simulink model "PuenteH_dcdc_CUESTION2"  (R2024b)
settings: Solver=ode23s  StartTime=0.0  StopTime=Ts*nciclos  FixedStep=fixedstep  MaxStep=Ts/ssamples  RelTol=Auto  AbsTol=1e-3
InitFcn:
  | Ts=1/fs;
values from neighbouring files (symbols this model uses):
  fs = 10e3    (= 10000)    [Cuestion2.m]    (also in DatosBasePuenteH.m)
  seleccion = 2    [Cuestion2.m]
  ssamples = 200    [Cuestion2.m]    (also in DatosBasePuenteH.m)
  Vcont = 2*D - 1    [Cuestion2.m]    (also in DatosBasePuenteH.m = -0.6)
libraries: simulink x2, spsMultimeterLib x2, spsControlledCurrentSourceLib x1, spsDCVoltageSourceLib x1, spsOnDelayLib x1, spsUniversalBridgeLib x1, spsVoltageMeasurementLib x1, sps_lib x1
settings Model: Creator=patrice  LastModifiedBy=Pablo
settings SolverCC: AutoScaleAbsTol=off  AlgebraicLoopSolver=TrustRegion
settings DataIOCC: SaveFormat=StructureWithTime  SignalLoggingSaveFormat=ModelDataLogs  ReturnWorkspaceOutputs=off  TimeSaveName=tiempo  SignalLoggingName=sigsOut
settings OptimizationCC: BlockReduction=off  BooleanDataType=off  ExpressionDepthLimit=2147483647  InitFltsAndDblsToZero=on  LifeSpan=inf
settings DebuggingCC: SaveWithParameterizedLinksMsg=none  UnderspecifiedInitializationDetection=Classic  MergeDetectMultiDrivingBlocksExec=none  SignalResolutionControl=TryResolveAllWithWarning  MultiTaskDSMMsg=warning  MultiTaskCondExecSysMsg=none  FcnCallInpInsideContextMsg=warning  StateNameClashWarn=warning  SFUnexpectedBacktrackingDiag=warning  SFNoUnconditionalDefaultTransitionDiag=warning  SFExecutionAtInitializationDiag=none  ArithmeticOperatorsInVariantConditions=warning
settings HardwareCC: ProdBitPerPointer=32  ProdBitPerSizeT=32  ProdBitPerPtrDiffT=32  ProdLargestAtomicFloat=None  ProdIntDivRoundTo=Undefined  ProdEndianess=Unspecified  ProdWordSize=32  ProdHWDeviceType=32-bit Generic  TargetUnknown=on
settings ModelReferenceCC: EnableRefExpFcnMdlSchedulingChecks=on  PropagateSignalLabelsOutOfModel=off
settings SFSimCC: SimUseLocalCustomCode=off  CustomCodeUndefinedFunction=UseInterfaceOnly
settings RTWCC: TemplateMakefile=grt_unix.tmf  RTWUseLocalCustomCode=off  GPUComputeCapability=3.5  DLArmComputeVersion=19.05
settings CodeAppCC: StateflowObjectComments=on
settings GRTTargetCC: TargetFcnLib=ansi_tfl_tmw.mat  TargetLangStandard=C89/C90 (ANSI)  CombineOutputUpdateFcns=off  GRTInterface=on
settings ConfigComp: CovMetricSettings=dw  CovSaveCumulativeToWorkspaceVar=on  CovSaveSingleToWorkspaceVar=on  CovExternalEMLEnable=off
settings SimscapeCC: SimscapeNormalizeSystem=off

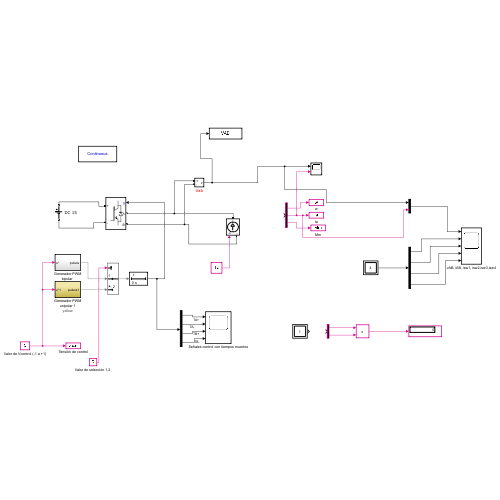
[thumbnail: Simulink's stored preview of the top-level diagram]
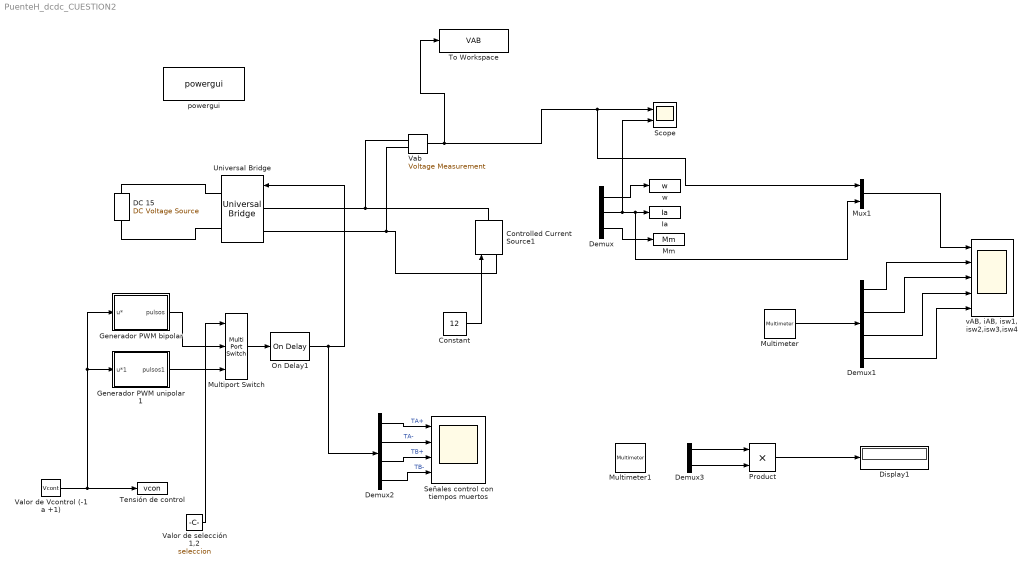
== system PuenteH_dcdc_CUESTION2 ==
  Constant : Constant  Value=12
  Controlled Current Source1 : spsControlledCurrentSourceLib/Controlled Current Source  Initialize=on  Source_Type=DC  Amplitude=12  Phase=0  Frequency=0  Measurements=Current
  DC 15 : spsDCVoltageSourceLib/DC Voltage Source  Amplitude=15  Measurements=Voltage
  Demux : Demux  Outputs=3
      settings: DisplayOption=none
  Demux1 : Demux
  Demux2 : Demux
  Demux3 : Demux  Outputs=2
  Display1 : Display
  "Generador PWM bipolar " : Subsystem
  Generador PWM unipolar 1 : Subsystem
      settings: AttributesFormatString=%<BackgroundColor>
  Ia : ToWorkspace  VariableName=Ia  SampleTime=-1
  Mm : ToWorkspace  VariableName=Mm  SampleTime=-1
  Multimeter : spsMultimeterLib/Multimeter  L=12  sel=[8 9 10 11]  yselected={}  Gain=[1 1 1 1]  OutputType=Complex  PlotAtSimulationStop=off  PhasorSimulation=off
  Multimeter1 : spsMultimeterLib/Multimeter  L=12  sel=7  yselected={}  Gain=1  OutputType=Complex  PlotAtSimulationStop=off  PhasorSimulation=off
  Multiport Switch : MultiPortSwitch  Inputs=2  SaturateOnIntegerOverflow=off  InputSameDT=off
  Mux1 : Mux  Inputs=2
  On Delay1 : spsOnDelayLib/On Delay  DelayType=On delay  delay=Tmuertos  ic=0  Ts=0
  Product : Product
  Scope : Scope  NumInputPorts=2
  Señales control con tiempos muertos : Scope  NumInputPorts=4
  Tensión de control : ToWorkspace  VariableName=vcon  SampleTime=-1
  To Workspace : ToWorkspace  VariableName=VAB  SaveFormat=Structure With Time  SampleTime=-1
  Universal Bridge : spsUniversalBridgeLib/Universal Bridge  Arms=2  SnubberResistance=1e5  SnubberCapacitance=inf  Device=IGBT / Diodes  Ron=1e-3  Lon=0  ForwardVoltages="[  0  0  ]"  ForwardVoltage=0  GTOparameters=[ 10e-6 , 20e-6 ]  IGBTparameters=[ 1e-6 , 2e-6 ]  Measurements=All voltages and currents  Measurements_2=None  converterType=Rectifier
  Vab : spsVoltageMeasurementLib/Voltage Measurement  PhasorSimulation=off  OutputType=Complex  PSBequivalent=0
  Valor de Vcontrol (-1 a +1) : Constant  Description=Aquí se ajusta el valor de la tensión de control, que tiene que estar entre -1 y +1 (valores de pico de la señal triangular)  Value=Vcont
  "Valor de selección 1,2 " : Constant  Value=seleccion
  powergui : sps_lib/powergui  SimulationMode=Continuous  SampleTime=Ts/ssamples  frequency=60  Iterations=50  frequencyindice=0  Pbase=100e6  ErrMax=1e-4  UnitsV=kV  UnitsW=MW  buscounter=0  FunctionMessages=off  echomessages=off  EnableUseOfTLC=off  CurrentSourceSwitches=off  DisableSnubberDevices=off  DisableRonSwitches=off  DisableVfSwitches=off  DisplayEquations=off  AutomaticDiscreteSolvers=off  SolverType=Tustin/Backward Euler (TBE)  Interpol=off  ExternalGateDelay=off  methode=off  Ts=100  x0status=blocks  SPID=off  SwTol=0  HookPort=off  NonlinearTolerance=1e-4  nMaxIteration=100  ContinueOnMaxIteration=off  RestoreLinks=warning  ResistiveCurrentMeasurement=off  Frange=[0:2:500]  Ylog=off  Xlog=on  ShowGrid=off  save=off  variable=ZData  structure=OutputPuente  ZoomFFT=on  StartTime=0.1  cycles=2  DisplayStyle=4  fundamental=10e3  FreqAxis=off  MaxFrequency=20*10e3  frequencyindicesteady=1  RmsSteady=1  display=off
  "vAB, iAB, isw1, isw2,isw3,isw4" : Scope  NumInputPorts=5
  w : ToWorkspace  VariableName=w  SampleTime=-1
  wires:
  "Generador PWM bipolar "/1(pulsos) -> Multiport Switch/2
  "Valor de selección 1,2 "/1 -> Multiport Switch/1
  Valor de Vcontrol (-1 a +1)/1 -> Tensión de control/1, Generador PWM unipolar 1/1(u*1), "Generador PWM bipolar "/1(u*)
  Demux/2 -> Scope/2, Mux1/2, Ia/1
  Demux/3 -> Mm/1
  Demux/1 -> w/1
  Vab/1 -> To Workspace/1, Mux1/1, Scope/1
  Multimeter/1 -> Demux1/1
  Mux1/1 -> "vAB, iAB, isw1, isw2,isw3,isw4"/1
  Demux1/1 -> "vAB, iAB, isw1, isw2,isw3,isw4"/2
  Demux1/2 -> "vAB, iAB, isw1, isw2,isw3,isw4"/3
  Demux1/3 -> "vAB, iAB, isw1, isw2,isw3,isw4"/4
  Demux1/4 -> "vAB, iAB, isw1, isw2,isw3,isw4"/5
  On Delay1/1 -> Demux2/1, Universal Bridge/1
  Multiport Switch/1 -> On Delay1/1
  Demux2/1 -> Señales control con tiempos muertos/1  "TA+"
  Demux2/2 -> Señales control con tiempos muertos/2  "TA-"
  Demux2/3 -> Señales control con tiempos muertos/3  "TB+"
  Demux2/4 -> Señales control con tiempos muertos/4  "TB-"
  Generador PWM unipolar 1/1(pulsos1) -> Multiport Switch/3
  Demux3/1 -> Product/1
  Demux3/2 -> Product/2
  Product/1 -> Display1/1
  Constant/1 -> Controlled Current Source1/1
  connections:
  Vab/LConn1 -- Controlled Current Source1/RConn1 -- Universal Bridge/LConn1
  Vab/LConn2 -- Controlled Current Source1/LConn1 -- Universal Bridge/LConn2
  DC 15/LConn1 -- Universal Bridge/RConn2
  Universal Bridge/RConn1 -- DC 15/RConn1

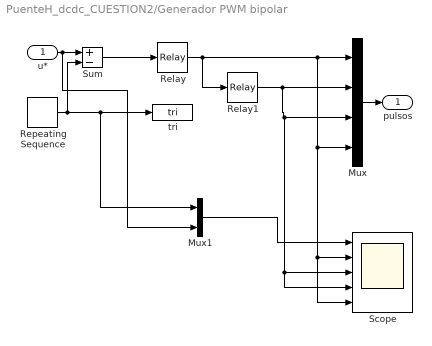
== system PuenteH_dcdc_CUESTION2/Generador PWM bipolar  ==
  u* : Inport
  Mux : Mux
  Mux1 : Mux  Inputs=2
  Relay : Relay  OnSwitchValue=0.01  OffSwitchValue=-0.01
  Relay1 : Relay  OnSwitchValue=0.51  OffSwitchValue=0.49  OnOutputValue=0  OffOutputValue=1
  Repeating Sequence : simulink/Sources/Repeating Sequence  rep_seq_t="[0 Ts/2  Ts]"  rep_seq_y=[-1 1 -1]
  Scope : Scope  NumInputPorts=5
  Sum : Sum  Inputs=+-  InputSameDT=on  SaturateOnIntegerOverflow=on  OutDataTypeStr=Inherit: Same as first input
  tri : ToWorkspace  VariableName=tri  SampleTime=-1
  pulsos : Outport
  wires:
  Sum/1 -> Relay/1
  Repeating Sequence/1 -> Sum/2, Mux1/1, tri/1
  u*/1 -> Mux1/2, Sum/1
  Relay1/1 -> Mux/2, Scope/4, Scope/3, Mux/3
  Mux/1 -> pulsos/1
  Mux1/1 -> Scope/1
  Relay/1 -> Relay1/1, Mux/1, Scope/2, Scope/5, Mux/4

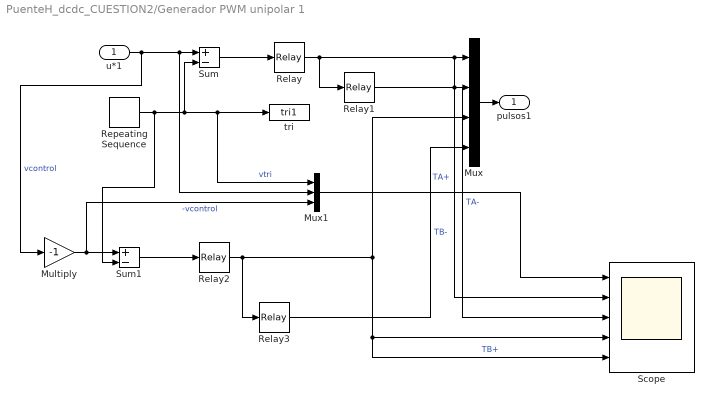
== system PuenteH_dcdc_CUESTION2/Generador PWM unipolar 1 ==
  u*1 : Inport
  Multiply : Gain  Gain=-1
  Mux : Mux
  Mux1 : Mux  Inputs=3
  Relay : Relay  OnSwitchValue=0.01  OffSwitchValue=-0.01
  Relay1 : Relay  OnSwitchValue=0.51  OffSwitchValue=0.49  OnOutputValue=0  OffOutputValue=1
  Relay2 : Relay  OnSwitchValue=0.01  OffSwitchValue=-0.01
  Relay3 : Relay  OnSwitchValue=0.51  OffSwitchValue=0.49  OnOutputValue=0  OffOutputValue=1
  Repeating Sequence : simulink/Sources/Repeating Sequence  rep_seq_t="[0 Ts/2  Ts]"  rep_seq_y=[-1 1 -1]
  Scope : Scope  NumInputPorts=5
  Sum : Sum  Inputs=+-  InputSameDT=on  SaturateOnIntegerOverflow=on  OutDataTypeStr=Inherit: Same as first input
  Sum1 : Sum  Inputs=+-  InputSameDT=on  SaturateOnIntegerOverflow=on  OutDataTypeStr=Inherit: Same as first input
  tri : ToWorkspace  VariableName=tri1  SampleTime=-1
  pulsos1 : Outport
  wires:
  Repeating Sequence/1 -> Sum1/2, Sum/2, Mux1/1, tri/1  "vtri"
  Mux/1 -> pulsos1/1
  u*1/1 -> Multiply/1, Mux1/2, Sum/1  "vcontrol"
  Sum/1 -> Relay/1
  Relay/1 -> Relay1/1, Scope/2, Mux/1  "TA+"
  Relay1/1 -> Scope/3, Mux/2  "TA-"
  Multiply/1 -> Mux1/3, Sum1/1  "-vcontrol"
  Sum1/1 -> Relay2/1
  Relay2/1 -> Relay3/1, Scope/5, Scope/4, Mux/3  "TB+"
  Relay3/1 -> Mux/4  "TB-"
  Mux1/1 -> Scope/1
